simulink model "InjCrv"  (R2018a)
settings: configuration reference "cs_ert" (kept outside this file)
settings Model: DataDictionary=InjCrv.sldd  Creator=zhoutinglin  LastModifiedBy=zhoutinglin

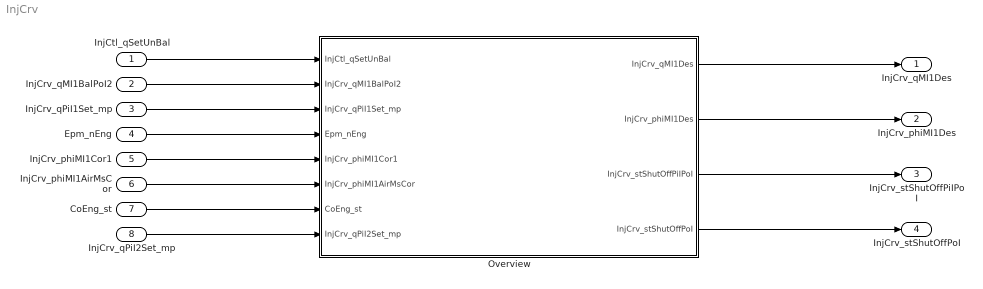
== system InjCrv ==
  InjCtl_qSetUnBal : Inport
  InjCrv_qMI1BalPoI2 : Inport  Port=2
  InjCrv_qPiI1Set_mp : Inport  Port=3
  Epm_nEng : Inport  Port=4
  InjCrv_phiMI1Cor1 : Inport  Port=5
  InjCrv_phiMI1AirMsCor : Inport  Port=6
  CoEng_st : Inport  Port=7
  InjCrv_qPiI2Set_mp : Inport  Port=8
  Overview : Subsystem
  InjCrv_qMI1Des : Outport
  InjCrv_phiMI1Des : Outport  Port=2
  InjCrv_stShutOffPiIPoI : Outport  Port=3
  InjCrv_stShutOffPoI : Outport  Port=4
  wires:
  InjCtl_qSetUnBal/1 -> Overview/1(InjCtl_qSetUnBal)
  InjCrv_qMI1BalPoI2/1 -> Overview/2(InjCrv_qMI1BalPoI2)
  InjCrv_qPiI1Set_mp/1 -> Overview/3(InjCrv_qPiI1Set_mp)
  Epm_nEng/1 -> Overview/4(Epm_nEng)
  InjCrv_phiMI1Cor1/1 -> Overview/5(InjCrv_phiMI1Cor1)
  InjCrv_phiMI1AirMsCor/1 -> Overview/6(InjCrv_phiMI1AirMsCor)
  CoEng_st/1 -> Overview/7(CoEng_st)
  InjCrv_qPiI2Set_mp/1 -> Overview/8(InjCrv_qPiI2Set_mp)
  Overview/1(InjCrv_qMI1Des) -> InjCrv_qMI1Des/1
  Overview/2(InjCrv_phiMI1Des) -> InjCrv_phiMI1Des/1
  Overview/3(InjCrv_stShutOffPiIPoI) -> InjCrv_stShutOffPiIPoI/1
  Overview/4(InjCrv_stShutOffPoI) -> InjCrv_stShutOffPoI/1

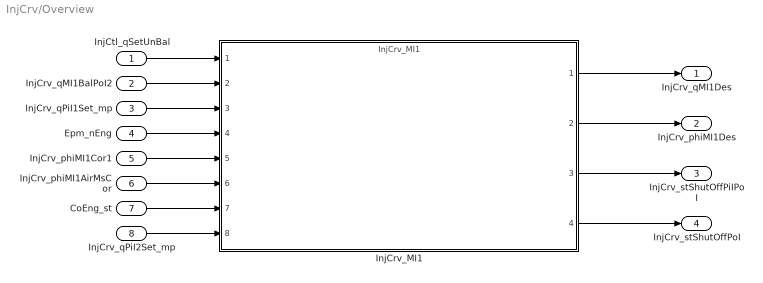
== system InjCrv/Overview ==
  InjCtl_qSetUnBal : Inport
  InjCrv_qMI1BalPoI2 : Inport  Port=2
  InjCrv_qPiI1Set_mp : Inport  Port=3
  Epm_nEng : Inport  Port=4
  InjCrv_phiMI1Cor1 : Inport  Port=5
  InjCrv_phiMI1AirMsCor : Inport  Port=6
  CoEng_st : Inport  Port=7
  InjCrv_qPiI2Set_mp : Inport  Port=8
  InjCrv_MI1 : ModelReference  ModelNameDialog=InjCrv_MI1  SimulationMode=Normal  ModelReferenceVersion=1.51
  InjCrv_qMI1Des : Outport
  InjCrv_phiMI1Des : Outport  Port=2
  InjCrv_stShutOffPiIPoI : Outport  Port=3
  InjCrv_stShutOffPoI : Outport  Port=4
  wires:
  InjCtl_qSetUnBal/1 -> InjCrv_MI1/1
  InjCrv_qMI1BalPoI2/1 -> InjCrv_MI1/2
  InjCrv_qPiI1Set_mp/1 -> InjCrv_MI1/3
  Epm_nEng/1 -> InjCrv_MI1/4
  InjCrv_phiMI1Cor1/1 -> InjCrv_MI1/5
  InjCrv_phiMI1AirMsCor/1 -> InjCrv_MI1/6
  CoEng_st/1 -> InjCrv_MI1/7
  InjCrv_qPiI2Set_mp/1 -> InjCrv_MI1/8
  InjCrv_MI1/1 -> InjCrv_qMI1Des/1
  InjCrv_MI1/2 -> InjCrv_phiMI1Des/1
  InjCrv_MI1/3 -> InjCrv_stShutOffPiIPoI/1
  InjCrv_MI1/4 -> InjCrv_stShutOffPoI/1
